simulink model "R_model"  (R2022b)
settings: Solver=VariableStepAuto  StartTime=0.0  StopTime=13  RelTol=1e-3
undefined symbols (not defined in the file): J, ke, km, L, R, target
settings Model: Creator=khanh  LastModifiedBy=Alex

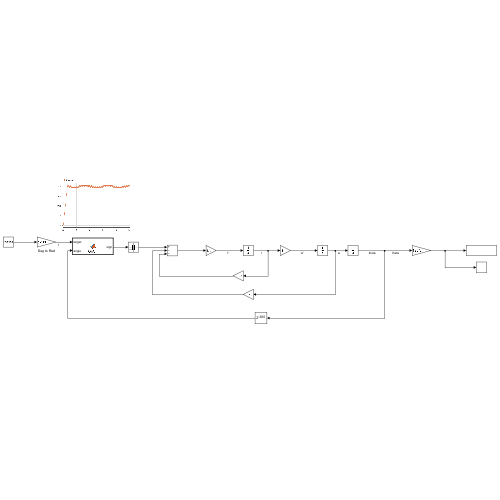
[thumbnail: Simulink's stored preview of the top-level diagram]
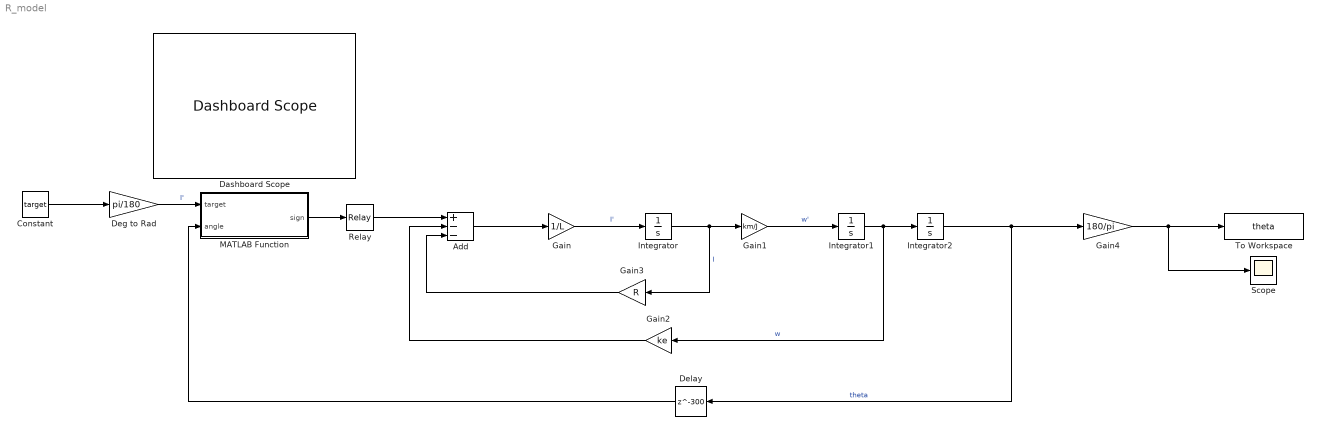
== system R_model ==
  Add : Sum  Inputs=+--
  Constant : Constant  Value=target
  Dashboard Scope : DashboardScope
  Deg to Rad : Gain  Gain=pi/180
  Delay : Delay  DelayLength=300  SampleTime=50e-6
  Gain : Gain  Gain=1/L
  Gain1 : Gain  Gain=km/J
  Gain2 : Gain  Gain=ke
  Gain3 : Gain  Gain=R
  Gain4 : Gain  Gain=180/pi
  Integrator : Integrator
  Integrator1 : Integrator
  Integrator2 : Integrator
  MATLAB Function : MATLAB Function  TreatAsAtomicUnit=on
  Relay : Relay  OnSwitchValue=0  OffSwitchValue=0  OnOutputValue=7.6  OffOutputValue=-7.6
  Scope : Scope
  To Workspace : ToWorkspace  VariableName=theta  SaveFormat=Timeseries  SampleTime=-1
  wires:
  Constant/1 -> Deg to Rad/1
  MATLAB Function/1(sign) -> Relay/1
  Relay/1 -> Add/1
  Add/1 -> Gain/1
  Gain/1 -> Integrator/1  "I'"
  Integrator/1 -> Gain3/1, Gain1/1  "I"
  Gain1/1 -> Integrator1/1  "w'"
  Integrator1/1 -> Gain2/1, Integrator2/1  "w"
  Integrator2/1 -> Delay/1, Gain4/1  "theta"
  Gain2/1 -> Add/2
  Gain3/1 -> Add/3
  Deg to Rad/1 -> MATLAB Function/1(target)  "I'"
  Gain4/1 -> Scope/1, To Workspace/1
  Delay/1 -> MATLAB Function/2(angle)

== matlab function R_model/MATLAB Function ==
  data: target input; sign output; angle input
function sign = OnOff(target, angle)
    sign = 0;
    if (target < angle)
        sign = -1;
    end
    if (target > angle)
        sign = 1;
    end
    if ( target == angle)
        sign = 0;
    end
